simulink model "computeDx"  (Simulink 7.7)
settings: Solver=FixedStepDiscrete  StartTime=0.0  StopTime=5  FixedStep=0.01  RelTol=1e-3
PreLoadFcn:
  | robotName = 'icubGazeboSim';
  | localName = 'SimulinkiCubGazeboSim';
InitFcn:
  | robotName = 'icubGazeboSim';
  | localName = 'SimulinkiCubGazeboSim';
libraries: WBCLibrary x7, simulink x1, utility x1
settings Model: Creator=iron  LastModifiedBy=iron

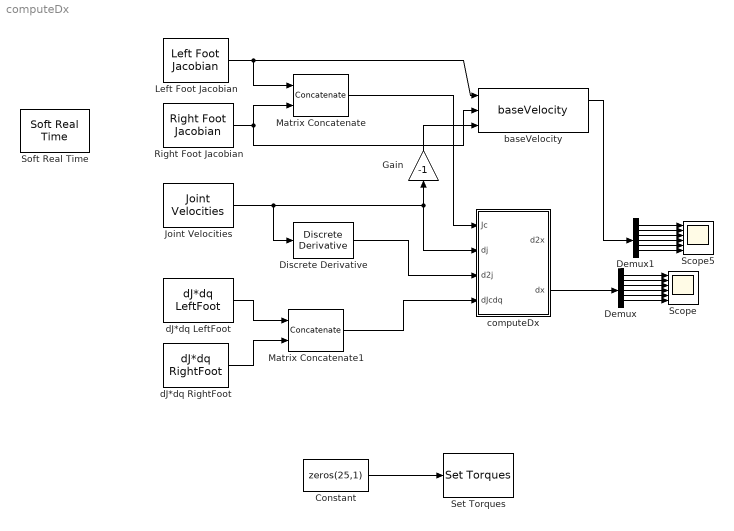
== system computeDx ==
  Constant : Constant  Value=zeros(25,1)
  Demux : Demux  Outputs=6
  Demux1 : Demux  Outputs=6
  Discrete Derivative : simulink/Discrete/Discrete Derivative  SystemSampleTime=-1  gainval=1.0  ICPrevScaledInput=0.0  OutMin=[]  OutMax=[]  OutDataType=fixdt(1, 16)  OutScaling=2^-10  DoSatur=off
  Gain : Gain  Gain=-1
  Joint Velocities : WBCLibrary/wholeBodyStates/Joint Velocities  SystemSampleTime=-1  robotName=robotName  localName=localName
  Left Foot Jacobian : WBCLibrary/wholeBodyModel/Jacobians/Left Foot Jacobian  SystemSampleTime=-1  robotName=robotName  localName=localName
  Matrix Concatenate : Concatenate  Mode=Multidimensional array
  Matrix Concatenate1 : Concatenate  Mode=Multidimensional array
  Right Foot Jacobian : WBCLibrary/wholeBodyModel/Jacobians/Right Foot Jacobian  SystemSampleTime=-1  robotName=robotName  localName=localName
  Scope : Scope  NumInputPorts=6
      settings: YMin=-0.0035~-0.0004~-0.0015~-0.0025~-0.03~-0.001  YMax=0.0005~0.0009~0.002~0.00025~0.005~0.00075
  Scope5 : Scope  NumInputPorts=6
      settings: YMin=-0.6~-0.00125~-0.025~-0.0025~-1.75~-0.0045  YMax=0.1~0.00125~0.225~0.0025~0.25~0.001  SaveName=ScopeData5
  Set Torques : WBCLibrary/wholeBodyActuators/Set Torques  SystemSampleTime=-1  val=6  robotName=robotName  localName=localName
  Soft Real Time : utility/Soft Real Time  x=1
  baseVelocity : WBCLibrary/Utilities/baseVelocity  SystemSampleTime=-1
  computeDx : Stateflow chart  TreatAsAtomicUnit=on
  dJ*dq LeftFoot : WBCLibrary/wholeBodyModel/Dynamics/dJ*dq LeftFoot  SystemSampleTime=-1  val=9  robotName=robotName  localName=localName
  dJ*dq RightFoot : WBCLibrary/wholeBodyModel/Dynamics/dJ*dq RightFoot  SystemSampleTime=-1  val=9  robotName=robotName  localName=localName
  wires:
  Left Foot Jacobian/1 -> Matrix Concatenate/1, baseVelocity/1
  Right Foot Jacobian/1 -> Matrix Concatenate/2, baseVelocity/2
  dJ*dq LeftFoot/1 -> Matrix Concatenate1/1
  dJ*dq RightFoot/1 -> Matrix Concatenate1/2
  Joint Velocities/1 -> Discrete Derivative/1, computeDx/2(dj), Gain/1
  Demux/1 -> Scope/1
  Demux/2 -> Scope/2
  Demux/3 -> Scope/3
  Demux/4 -> Scope/4
  Demux/5 -> Scope/5
  Demux/6 -> Scope/6
  Discrete Derivative/1 -> computeDx/3(d2j)
  Matrix Concatenate1/1 -> computeDx/4(dJcdq)
  Demux1/1 -> Scope5/1
  Demux1/2 -> Scope5/2
  Demux1/3 -> Scope5/3
  Demux1/4 -> Scope5/4
  Demux1/5 -> Scope5/5
  Demux1/6 -> Scope5/6
  Gain/1 -> baseVelocity/3
  Matrix Concatenate/1 -> computeDx/1(Jc)
  Constant/1 -> Set Torques/1
  baseVelocity/1 -> Demux1/1
  computeDx/2(dx) -> Demux/1

== matlab function computeDx ==
  data: d2x output double; dx output double; Jc input double; dj input double; d2j input double; dJcdq input double
function [d2x, dx] = fcn(Jc, dj, d2j, dJcdq)

% Francesco Nori
% Genova 6 Marzo 2014
% CODYCO project
%
% This code computes the torques tau necessary to obtain a desired
% acceleration d2q in a kinematic chain with contacts. These 
% computations are described in (DelPrete,2013) Ph.D. thesis
% and can be found also in [Aghili 2005; Righetti et al. 2011]. It can
% be shown that:
%
% tau = pinv(Nc' S') Nc (M d2q  + h)  
%
% with Nc = (I-pinv(Jc)Jc) and the constraints being described as:
%
% Jc dq = 0
%
% Jc d2q + dJcdq= 0

Jx = Jc(:,1:6);
Jj = Jc(:,7:end);
d2x = pinv(Jx)*(-Jj*d2j+dJcdq);
dx = pinv(Jx)*(-Jj*dj);
